simulink model "QuarterCarModel1"  (R2023b)
settings: Solver=VariableStepAuto  StartTime=0.0  StopTime=10.0  RelTol=1e-3
values from neighbouring files (symbols this model uses):
  d = 50    [QuarterCarWrapperScript.m]
  h_s = 1    [QuarterCarWrapperScript.m]
  h_t = 0    [QuarterCarWrapperScript.m]
  h_u = 0.5    [QuarterCarWrapperScript.m]
  k_s = 50000    [QuarterCarWrapperScript.m]
  k_t = 127000    [QuarterCarWrapperScript.m]
  m_s = 50    [QuarterCarWrapperScript.m]
  m_t = 4    [QuarterCarWrapperScript.m]
settings Model: Creator=emily  LastModifiedBy=emily

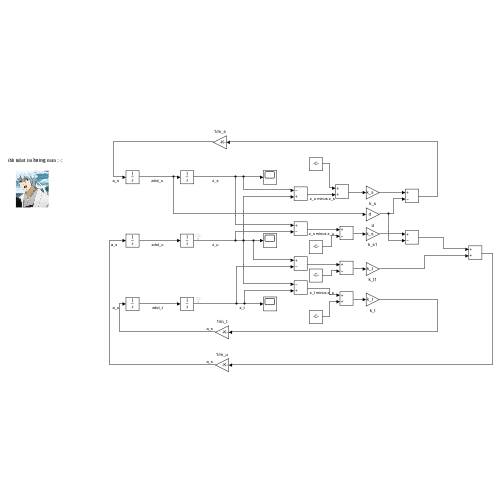
[thumbnail: Simulink's stored preview of the top-level diagram]
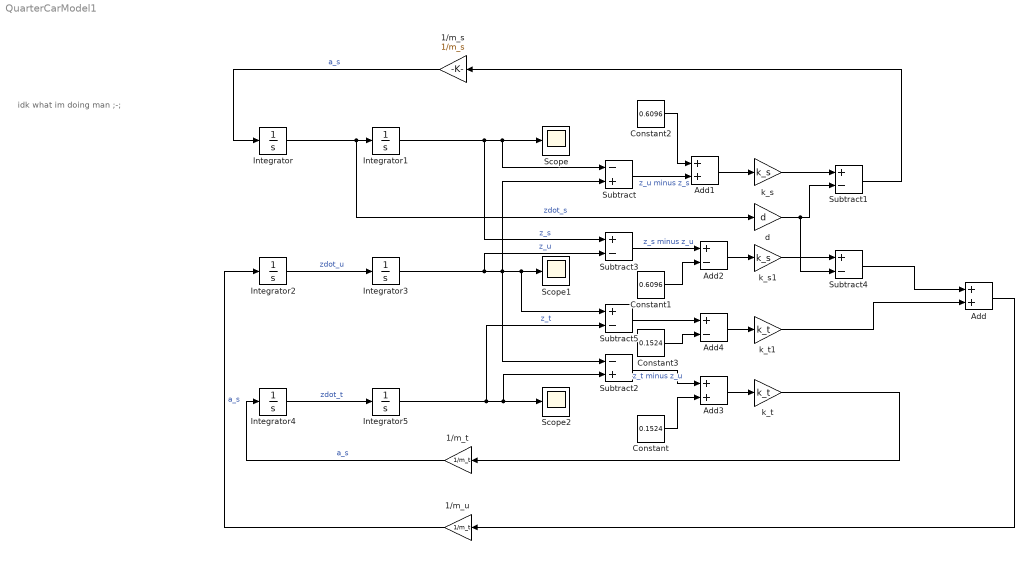
== system QuarterCarModel1 ==
  note: idk what im doing man ;-;
  1/m_s : Gain  Gain=1/m_s
  1/m_t : Gain  Gain=1/m_t
  1/m_u : Gain  Gain=1/m_t
  Add : Sum
  Add1 : Sum
  Add2 : Sum  Inputs=+-
  Add3 : Sum
  Add4 : Sum  Inputs=+-
  Constant : Constant  Value=0.1524
  Constant1 : Constant  Value=0.6096
  Constant2 : Constant  Value=0.6096
  Constant3 : Constant  Value=0.1524
  Integrator : Integrator
  Integrator1 : Integrator  InitialCondition=h_s
  Integrator2 : Integrator
  Integrator3 : Integrator  InitialCondition=h_u
  Integrator4 : Integrator
  Integrator5 : Integrator  InitialCondition=h_t
  Scope : Scope
  Scope1 : Scope
  Scope2 : Scope
  Subtract : Sum  Inputs=-+
  Subtract{1,3..5} (4 alike) : Sum  Inputs=+-
  Subtract2 : Sum  Inputs=-+
  d : Gain  Gain=d
  k_s : Gain  Gain=k_s
  k_s1 : Gain  Gain=k_s
  k_t : Gain  Gain=k_t
  k_t1 : Gain  Gain=k_t
  wires:
  Integrator1/1 -> Subtract3/1, Scope/1, Subtract/1  "z_s"
  Integrator/1 -> d/1, Integrator1/1  "zdot_s"
  1/m_s/1 -> Integrator/1  "a_s"
  Integrator2/1 -> Integrator3/1  "zdot_u"
  Integrator3/1 -> Subtract3/2, Subtract2/1, Subtract5/1, Scope1/1, Subtract/2  "z_u"
  Subtract/1 -> Add1/2  "z_u minus z_s"
  k_s/1 -> Subtract1/1
  d/1 -> Subtract4/2, Subtract1/2
  Subtract1/1 -> 1/m_s/1
  Integrator5/1 -> Subtract5/2, Scope2/1, Subtract2/2  "z_t"
  Integrator4/1 -> Integrator5/1  "zdot_t"
  Subtract2/1 -> Add3/1  "z_t minus z_u"
  1/m_t/1 -> Integrator4/1  "a_s"
  k_t/1 -> 1/m_t/1
  Add/1 -> 1/m_u/1
  1/m_u/1 -> Integrator2/1  "a_s"
  Add1/1 -> k_s/1
  Constant2/1 -> Add1/1
  Subtract3/1 -> Add2/1  "z_s minus z_u"
  Constant1/1 -> Add2/2
  Add2/1 -> k_s1/1
  Subtract4/1 -> Add/1
  Add3/1 -> k_t/1
  Constant/1 -> Add3/2
  Subtract5/1 -> Add4/1
  Constant3/1 -> Add4/2
  Add4/1 -> k_t1/1
  k_s1/1 -> Subtract4/1
  k_t1/1 -> Add/2
